simulink model "c_citation"  (R2020a)
settings: Solver=ode5  StartTime=0.0  StopTime=inf  FixedStep=0.01  RelTol=1e-3
InitFcn:
  | load('simulation_parameters');
values from neighbouring files (symbols this model uses):
  chord = 1.991    [citdata.mat]
  cv1 = 20000    [gear_params.m]
  cv2 = cv1    (= 20000)    [gear_params.m]
  cv3 = 4000    [gear_params.m]
  cv4 = 20000    [gear_params.m]
  deltagmax1 = 0.25    [gear_params.m]
  deltagmax2 = deltagmax1    (= 0.25)    [gear_params.m]
  deltagmax3 = 0.24    [gear_params.m]
  deltagmax4 = 0.02    [gear_params.m]
  ealphag = [0  0.2618  0.6981; 1  1.3  0.8]    [citdata.mat]
  ealphas = [0  0.2618  0.6981; 0.157  0.157  0.175]    [citdata.mat]
  g0 = 9.80665    [ac_genrl.mat]
  hDME = 0    [ac_genrl.mat]
  hGS = 0    [ac_genrl.mat]
  kt1 = 525020    [gear_params.m]
  kt2 = kt1    (= 525020)    [gear_params.m]
  kt3 = 457050    [gear_params.m]
  lh = 5.53    [citdata.mat]
  matbuaf = [0  -0.1745  0.4363; 0  -0.1  -0.1; 0.6981  -0.1  -0.1]    [citdata.mat]
  matdaf = [0 0 0.2618 0.6981 0.734842105263 0.771584210526 0.808326315789 0.845068421053 0.881810526316 0.918552631579 0.955294736842 0.992036842105 ... (529 elements, 23x23)]    [citdata.mat]
  matdam = [0 0.05 0.15 0.25 0.35 0.45 0.55 0.65 0.75 0.803571428571 0.857142857143 0.910714285714 ... (529 elements, 23x23)]    [citdata.mat]
  matdbbf = [0 0 0.6981 0.74464 0.79118 0.83772 0.88426 0.9308 0.97734 1.02388 1.07042 1.11696 ... (324 elements, 18x18)]    [citdata.mat]
  matdeaf = [0 0 0.2618 0.6981 0.734842105263 0.771584210526 0.808326315789 0.845068421053 0.881810526316 0.918552631579 0.955294736842 0.992036842105 ... (529 elements, 23x23)]    [citdata.mat]
  matdgaf = [0 0 0.2618 0.6981 -0.1745 -0.0175 -0.008 -0.009 0.4363 -0.0175 -0.008 -0.009 ... (16 elements, 4x4)]    [citdata.mat]
  matdqaf = [0 0 0.2618 0.6981 0.734842105263 0.771584210526 0.808326315789 0.845068421053 0.881810526316 0.918552631579 0.955294736842 0.992036842105 ... (529 elements, 23x23)]    [citdata.mat]
  matduaf = [0 0 0.2618 0.6981 0.734842105263 0.771584210526 0.808326315789 0.845068421053 0.881810526316 0.918552631579 0.955294736842 0.992036842105 ... (529 elements, 23x23)]    [citdata.mat]
  matdwaw = [0 0 0.1745 0.3491 0.5236 0.6458 1.2916 -0.1745 0 0.0018 0.0046 0.0088 ... (49 elements, 7x7)]    [citdata.mat]
  matedhr = [0 1 1 0.71 2 0.51 3 0.34 5 0.12 7.5 0.03 ... (20 elements, 2x10)]    [citdata.mat]
  mateif = [0  0.2618  0.6981; 0  -0.075  -0.075]    [citdata.mat]
  matelhr = [0 1 1 0.95 2 0.91 3 0.84 5 0.71 7.5 0.35 ... (20 elements, 2x10)]    [citdata.mat]
  matemhr = [0 1 1 0.9 2 0.8 3 0.7 5 0.5 7.5 0.25 ... (20 elements, 2x10)]    [citdata.mat]
  matemv1 = [0  90  100; 0  1  1]    [citdata.mat]
  matemv2 = [20  75  90; 0  1  1]    [citdata.mat]
  matemve = [0  90  100; 0  1  1]    [citdata.mat]
  matetam = [0  -0.1745  0.4363; 0  -0.04  -0.04; 1  -0.04  -0.04]    [citdata.mat]
  mateuaf = [0 0 0.6981 0.733005 0.76791 0.802815 0.83772 0.872625 0.90753 0.942435 0.97734 1.012245 ... (529 elements, 23x23)]    [citdata.mat]
  matfaaf = [0 0 0.2618 0.6981 0.734842105263 0.771584210526 0.808326315789 0.845068421053 0.881810526316 0.918552631579 0.955294736842 0.992036842105 ... (529 elements, 23x23)]    [citdata.mat]
  matfaxl = [0.15  0.35; 1  1]    [citdata.mat]
  matibaf = [0 0 0.2618 0.6981 -0.2 -0.119 -0.117 -0.108 0.3 -0.059 -0.052 -0.038 ... (16 elements, 4x4)]    [citdata.mat]
  matibb = [0 0 0.2618 1.571 3.142 -0.2 0 0 0.074 0.124 0 0 ... (50 elements, 5x10)]    [citdata.mat]
  matibmh = [0 0 15000 17142.8571429 19285.7142857 21428.5714286 23571.4285714 25714.2857143 27857.1428571 30000 0 0 ... (100 elements, 10x10)]    [citdata.mat]
  matipaf = [0  -0.1745  0.4363; 0  -0.44  -0.44; 0.6981  -0.44  -0.44]    [citdata.mat]
  matipmh = [0 0 15000 17142.8571429 19285.7142857 21428.5714286 23571.4285714 25714.2857143 27857.1428571 30000 0 0 ... (100 elements, 10x10)]    [citdata.mat]
  matiraf = [0 0 0.2618 0.6981 -0.2 0.05 -0.03 0.01 0.3 0.3 0.37 0.41 ... (16 elements, 4x4)]    [citdata.mat]
  matiuaf = [0  -0.2  0.3; 0  0.052  -0.003; 0.6981  0.052  -0.003]    [citdata.mat]
  matiwaf = [0  -0.1745  0.4363; 0  -0.185  -0.185; 0.6981  -0.185  -0.185]    [citdata.mat]
  matlaf = [0 0 0.2618 0.6981 0.734842105263 0.771584210526 0.808326315789 0.845068421053 0.881810526316 0.918552631579 0.955294736842 0.992036842105 ... (529 elements, 23x23)]    [citdata.mat]
  matlam = [0 0.05 0.15 0.25 0.35 0.45 0.55 0.65 0.75 0.803571428571 0.857142857143 0.910714285714 ... (529 elements, 23x23)]    [citdata.mat]
  matleaf = [0 0 0.2618 0.6981 0.734842105263 0.771584210526 0.808326315789 0.845068421053 0.881810526316 0.918552631579 0.955294736842 0.992036842105 ... (529 elements, 23x23)]    [citdata.mat]
  matleam = [0  -0.1745  0.4363; 0  0.58  0.58; 1  0.58  0.58]    [citdata.mat]
  matlgaf = [0 0 0.2618 0.6981 -0.1745 0.045 0.105 0.14 0.4363 0.045 0.105 0.14 ... (16 elements, 4x4)]    [citdata.mat]
  matlqaf = [0 0 0.2618 0.6981 0.734842105263 0.771584210526 0.808326315789 0.845068421053 0.881810526316 0.918552631579 0.955294736842 0.992036842105 ... (529 elements, 23x23)]    [citdata.mat]
  matluaf = [0 0 0.2618 0.6981 0.734842105263 0.771584210526 0.808326315789 0.845068421053 0.881810526316 0.918552631579 0.955294736842 0.992036842105 ... (529 elements, 23x23)]    [citdata.mat]
  matmaaf = [0 0 0.2618 0.6981 0.734842105263 0.771584210526 0.808326315789 0.845068421053 0.881810526316 0.918552631579 0.955294736842 0.992036842105 ... (484 elements, 22x22)]    [citdata.mat]
  matmaam = [0 0.05 0.15 0.25 0.35 0.45 0.55 0.65 0.75 0.803571428571 0.857142857143 0.910714285714 ... (484 elements, 22x22)]    [citdata.mat]
  matmaf = [0 0 0.2618 0.6981 0.734842105263 0.771584210526 0.808326315789 0.845068421053 0.881810526316 0.918552631579 0.955294736842 0.992036842105 ... (529 elements, 23x23)]    [citdata.mat]
  matmam = [0 0.05 0.15 0.25 0.35 0.45 0.55 0.65 0.75 0.803571428571 0.857142857143 0.910714285714 ... (529 elements, 23x23)]    [citdata.mat]
  matmbbf = [0 0 0.6981 0.74464 0.79118 0.83772 0.88426 0.9308 0.97734 1.02388 1.07042 1.11696 ... (324 elements, 18x18)]    [citdata.mat]
  matmeaf = [0 0 0.2618 0.6981 0.734842105263 0.771584210526 0.808326315789 0.845068421053 0.881810526316 0.918552631579 0.955294736842 0.992036842105 ... (529 elements, 23x23)]    [citdata.mat]
  matmeam = [0 0 1 1.05 1.1 1.15 1.2 1.25 1.3 1.35 1.4 1.45 ... (529 elements, 23x23)]    [citdata.mat]
  matmgaf = [0 0 0.2618 0.6981 -0.1745 -0.01 -0.024 -0.035 0.4363 -0.01 -0.024 -0.035 ... (16 elements, 4x4)]    [citdata.mat]
  matmqaf = [0 0 0.2618 0.6981 0.734842105263 0.771584210526 0.808326315789 0.845068421053 0.881810526316 0.918552631579 0.955294736842 0.992036842105 ... (529 elements, 23x23)]    [citdata.mat]
  matmrbr = [0  0  0.5236; 0  0  0; 0.384  0.001  0.001]    [citdata.mat]
  matnbab = [0 0 0.2618 1.571 3.142 -0.2 0 0 -0.0199 -0.1049 0 0 ... (25 elements, 5x5)]    [citdata.mat]
  matnbaf = [0  -0.2  0.3; 0  0.105  0.18; 0.6981  0.105  0.18]    [citdata.mat]
  matnbmh = [0 0 15000 17142.8571429 19285.7142857 21428.5714286 23571.4285714 25714.2857143 27857.1428571 30000 0 0 ... (100 elements, 10x10)]    [citdata.mat]
  matnpaf = [0 0 0.2618 0.6981 -0.2 0.03 0.03 0.05 0.3 -0.12 -0.12 -0.2 ... (16 elements, 4x4)]    [citdata.mat]
  matnpmh = [0 0 15000 17142.8571429 19285.7142857 21428.5714286 23571.4285714 25714.2857143 27857.1428571 30000 0 0 ... (100 elements, 10x10)]    [citdata.mat]
  matnraf = [0  -0.1745  0.4363; 0  -0.21  -0.21; 0.6981  -0.21  -0.21]    [citdata.mat]
  matnuaf = [0  -0.1745  0.4363; 0  -0.101  -0.101; 0.6981  -0.101  -0.101]    [citdata.mat]
  matnwaf = [0 0 0.2618 0.6981 -0.2 -0.02 -0.037 -0.049 0.3 0.03 0.043 0.036 ... (16 elements, 4x4)]    [citdata.mat]
  matnwmh = [0 0 15000 17142.8571429 19285.7142857 21428.5714286 23571.4285714 25714.2857143 27857.1428571 30000 0 0 ... (100 elements, 10x10)]    [citdata.mat]
  matqlaf = [0  -0.1745  0.4363; 0  -1  -1; 0.6981  -1  -1]    [citdata.mat]
  matquaf = [0 0 0.6981 0.733005 0.76791 0.802815 0.83772 0.872625 0.90753 0.942435 0.97734 1.012245 ... (529 elements, 23x23)]    [citdata.mat]
  matqxl = [0.15  0.35; 1  1]    [citdata.mat]
  matqxm = [0.15  0.35; 1  1]    [citdata.mat]
  matrtam = [0  -0.1745  0.4363; 0  0.011  0.011; 1  0.011  0.011]    [citdata.mat]
  matruaf = [0  -0.1745  0.4363; 0  0.2  0.2; 0.6981  0.2  0.2]    [citdata.mat]
  matrumh = [0 0 15000 17142.8571429 19285.7142857 21428.5714286 23571.4285714 25714.2857143 27857.1428571 30000 0 0 ... (100 elements, 10x10)]    [citdata.mat]
  matuut = [0  0.5  1; 0  1.35  1]    [citdata.mat]
  matwtam = [0  -0.1745  0.4363; 0  0.011  0.011; 1  0.011  0.011]    [citdata.mat]
  matybab = [0 0 0.2618 1.571 3.142 -0.2 0 0 0.34 0.75 0 0 ... (25 elements, 5x5)]    [citdata.mat]
  matybaf = [0  -0.1745  0.4363; 0  -0.75  -0.75; 0.6981  -0.75  -0.75]    [citdata.mat]
  matyraf = [0  -0.1745  0.4363; 0  0.85  0.85; 0.6981  0.85  0.85]    [citdata.mat]
  matyuaf = [0  -0.1745  0.4363; 0  0.23  0.23; 0.6981  0.23  0.23]    [citdata.mat]
  matywaf = [0  -0.1745  0.4363; 0  -0.04  -0.04; 0.6981  -0.04  -0.04]    [citdata.mat]
  murol = 0.03*10    (= 0.3)    [gear_params.m]
  P1 = 2000    [gear_params.m]
  P2 = P1    (= 2000)    [gear_params.m]
  P3 = 2550    [gear_params.m]
  P4 = 40000    [gear_params.m]
  psiLOC = 0    [ac_genrl.mat]
  pstat0 = 101325    [ac_genrl.mat]
  S = 24.99    [citdata.mat]
  span = 13.325    [citdata.mat]
  T0 = 288.15    [ac_genrl.mat]
  tilteng = [0 0]    [citdata.mat]
  toweng = [0 0]    [citdata.mat]
  vdommyr37 = [0  0.2618  0.6981; 0  0.025  0]    [citdata.mat]
  vdommyr38 = [0  0.2618  0.6981; -0.01  0  -0.01]    [citdata.mat]
  Vw915 = 0    [initcit.m]
  winddir = 45*(pi/180)    (= 0.785398163397)    [initcit.m]
  xcgref = 6.5    [citdata.mat]
  xDME = 0    [ac_genrl.mat]
  xeng = [8.407 8.407]    [citdata.mat]
  xGS = 0    [ac_genrl.mat]
  xiacc = 3.2    [ac_genrl.mat]
  xl1 = xcg-6.858    [gear_params.m]
  xl2 = xcg-6.858    [gear_params.m]
  xl3 = xcg-2.0752    [gear_params.m]
  xl4 = xcg-12.742    [gear_params.m]
  xLOC = 0    [ac_genrl.mat]
  ycgref = 0    [citdata.mat]
  yDME = 0    [ac_genrl.mat]
  yeng = [3 -3]    [citdata.mat]
  yGS = 0    [ac_genrl.mat]
  yiacc = 0    [ac_genrl.mat]
  yl1 = 1.918    [gear_params.m]
  yl2 = -1.918    [gear_params.m]
  yl3 = 0    [gear_params.m]
  ... (+9 more)
undefined symbols (not defined in the file or in its folder): Deng, massinit, matff, matn1d, matn2d, matthr, u0, ut0, x0, xt0
(part 1 of 5)
settings Model: ExtModeTrigMode=oneshot  ExtModeArmWhenConnect=off  Creator=laurensvaneykeren  LastModifiedBy=kdally
settings DataIOCC: SaveFormat=Array  SignalLoggingSaveFormat=ModelDataLogs  ReturnWorkspaceOutputs=off  SignalLoggingName=sigsOut
settings OptimizationCC: DefaultParameterBehavior=Inlined  UseDivisionForNetSlopeComputation=on  UseFloatMulNetSlope=on  InlineInvariantSignals=on  EnhancedBackFolding=on  PassReuseOutputArgsAs=Individual arguments  ExpressionDepthLimit=2147483647  ZeroExternalMemoryAtStartup=off  ZeroInternalMemoryAtStartup=off  NoFixptDivByZeroProtection=on  EfficientFloat2IntCast=on  OptimizeBlockOrder=speed  DifferentSizesBufferReuse=on  OptimizationCustomize=off  EfficientTunableParamExpr=on
settings DebuggingCC: ReadBeforeWriteMsg=EnableAllAsError  WriteAfterWriteMsg=EnableAllAsError  WriteAfterReadMsg=EnableAllAsError  SaveWithParameterizedLinksMsg=none  SignalResolutionControl=TryResolveAllWithWarning  MultiTaskRateTransMsg=warning  IntegerOverflowMsg=error  ParameterTunabilityLossMsg=error  FcnCallInpInsideContextMsg=warning  UniqueDataStoreMsg=error  StateNameClashWarn=warning  NonBusSignalsTreatedAsBus=error  SFInvalidInputDataAccessInChartInitDiag=error  SFTransitionOutsideNaturalParentDiag=error  SFUnreachableExecutionPathDiag=error  SFUndirectedBroadcastEventsDiag=error  SFExecutionAtInitializationDiag=none  IntegerSaturationMsg=error  ArithmeticOperatorsInVariantConditions=warning
settings HardwareCC: ProdBitPerLong=64  ProdHWDeviceType=Intel->x86-64 (Mac OS X)  TargetBitPerLong=64  TargetBitPerPointer=64  TargetBitPerSizeT=64  TargetBitPerPtrDiffT=64  TargetLongLongMode=on  TargetIntDivRoundTo=Zero  TargetEndianess=LittleEndian  TargetWordSize=64  TargetHWDeviceType=MATLAB Host  ProdEqTarget=off
settings SFSimCC: SimUseLocalCustomCode=off  MATLABDynamicMemAlloc=off  CustomCodeUndefinedFunction=UseInterfaceOnly
settings SFSimCC: SimCustomSourceCode=|
  | ac_axes.c
  | ac_atmos.c
settings RTWCC: SystemTargetFile=ert.tlc  GenCodeOnly=on  TemplateMakefile=ert_default_tmf  GenerateReport=on  RTWUseLocalCustomCode=off  BuildConfiguration=Faster Runs  IncludeHyperlinkInReport=on  LaunchReport=on  GenerateTraceInfo=on  GenerateTraceReport=on  GenerateTraceReportSl=on  GenerateTraceReportSf=on  GenerateTraceReportEml=on  GenerateCodeMetricsReport=on  CheckMdlBeforeBuild=Warning
settings CodeAppCC: ForceParamTrailComments=on  IgnoreCustomStorageClasses=off  OperatorAnnotations=on  SimulinkDataObjDesc=on  SFDataObjDesc=on  CustomSymbolStrGlobalVar=rt$N$M  CustomSymbolStrType=$N$M  CustomSymbolStrFcn=$N$M$F  CustomSymbolStrMacro=$N$M  InsertBlockDesc=on
settings ERTTargetCC: TargetLangStandard=C99 (ISO)  GenerateSampleERTMain=on  SupportAbsoluteTime=off  SupportComplex=off  SupportContinuousTime=on  SupportNonInlinedSFcns=on  InlinedParameterPlacement=NonHierarchical  ERTCustomFileTemplate=example_file_process.tlc
settings ConfigComp: CovMetricSettings=dw  CovHtmlReporting=on  CovSaveCumulativeToWorkspaceVar=on  CovSaveSingleToWorkspaceVar=on  CovExternalEMLEnable=off

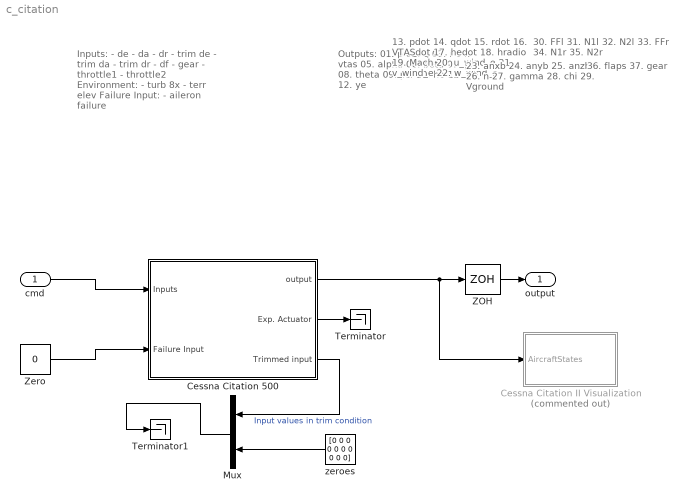
== system c_citation ==
  note: Inputs:
      |   - de
      |   - da
      |   - dr
      |   - trim de
      |   - trim da
      |   - trim dr
      |   - df
      |   - gear
      |   - throttle1
      |   - throttle2
      | Environment:
      |   - turb 8x
      |   - terr elev
      | Failure Input:
      |   - aileron failure
  note: Outputs:
      |   01. p
      |   02. q
      |   03. r
      |   04. vtas
      |   05. alpha
      |   06. beta
      |   07. phi
      |   08. theta
      |   09. psi
      |   10. he
      |   11. xe
      |   12. ye
  note: 13. pdot
      |   14. qdot
      |   15. rdot
      |   16. VTASdot
      |   17. hedot
      |   18. hradio
      |   19. Mach
      |   20. u_wind_e
      |   21. v_wind_e
      |   22. w_wind_e
  note: 23. anxb
      |   24. anyb
      |   25. anzb
      |   26. n
      |   27. gamma
      |   28. chi
      |   29. Vground
  note: 30. FFl
      |   31. N1l
      |   32. N2l
      |   33. FFr
      |   34. N1r
      |   35. N2r
  note: 36. flaps
      |   37. gear
  cmd : Inport  PortDimensions=10
  Cessna Citation 500 : Subsystem  mask(Citation Aircraft Model){trimdatafile=example.tri}
      mask prompts: trimdatafile "Trim Condition"
      mask init:
      | initcit;
      mask Display:
      | image(imread('Citation.jpg'))
      | port_label('input', 1, 'Inputs')
      | port_label('input', 2, 'Environment')
      | port_label('input', 3, 'Failure Input')
      | port_label('output', 1, 'Outputs')
      | port_label('output', 2, 'Exp. Actuator')
      | port_label('output', 3, 'Trim inputs')
  Cessna Citation II Visualization : Subsystem  Commented=on
  Mux : Mux  Inputs=2
  Terminator : Terminator
  Terminator1 : Terminator
  ZOH : ZeroOrderHold  SampleTime=-1
  Zero : Constant  Value=0  OutDataTypeStr=Inherit: Inherit via back propagation
  zeroes : Constant  Value=[0 0 0 0 0 0 0 0 0 0]  SampleTime=-1
  output : Outport  VectorParamsAs1DForOutWhenUnconnected=off
  wires:
  Cessna Citation 500/1(output) -> ZOH/1, Cessna Citation II Visualization/1(AircraftStates)
  Cessna Citation 500/3(Trimmed input) -> Mux/1  "Input values in trim condition"
  Cessna Citation 500/2(Exp. Actuator) -> Terminator/1
  cmd/1 -> Cessna Citation 500/1(Inputs)
  zeroes/1 -> Mux/2
  ZOH/1 -> output/1
  Zero/1 -> Cessna Citation 500/2(Failure Input)
  Mux/1 -> Terminator1/1

== system c_citation/Cessna Citation 500 ==
  note: p
      | q
      | r
      | vtas
      | alpha
      | beta
      | phi
      | theta
      | psi
      | he
      | xe
      | ye
  note: de
      | da
      | dr
      | dte
      | dta
      | dtr
      | df
      | gear
      | pla1
      | pla2
  note: pdot
      | qdot
      | rdot
      | VTASdot
      | hedot
  note: hradio
      | Mach
      | u_wind_e
      | v_wind_e
      | w_wind_e
  note: anxb
      | anyb
      | anzb
      | n
  note: gamma
      | chi
      | Vground
  note: turb 8x
      | terr_elev
  note: flaps
      | gear
  note: de
      | da
      | dr
      | dte
      | dta
      | dtr
      | df
      | gear
      | pla1
      | pla2
  note: FFl
      | N1l
      | N2l
      | FFr
      | N1r
      | N2r
  Inputs : Inport
  Failure Input : Inport  Port=2
  Actuators : Subsystem
  Citation model DASMAT : Subsystem
  Controllers : Subsystem
  Demux4 : Demux  Outputs=[8 2]
      settings: DisplayOption=none
  Mux1 : Mux  Inputs=7
  Mux2 : Mux  Inputs=2
  Terminator : Terminator
  Vector Concatenate : Concatenate  NumInputs=9
  Zero1 : Constant  Value=0  OutDataTypeStr=Inherit: Inherit via back propagation
  trim conditions : Subsystem
  ua sel : Selector  IndexOptions=Index vector (dialog)  Indices=[5 6]  OutputSizes=1
  xdot sel : Selector  IndexOptions=Index vector (dialog)  Indices=[1 2 3 4 10]  OutputSizes=1
  yacc sel : Selector  IndexOptions=Index vector (dialog)  Indices=[4 5 6 15]  OutputSizes=1
  yair sel : Selector  IndexOptions=Index vector (dialog)  Indices=[6 9 22 23 24]  OutputSizes=1
  yfp sel : Selector  IndexOptions=Index vector (dialog)  Indices=[1 2 15]  OutputSizes=1
  ypp sel : Selector  IndexOptions=Index vector (dialog)  Indices=[2 3 4 13 14 15]  OutputSizes=1
  output : Outport  PortDimensions=12  VectorParamsAs1DForOutWhenUnconnected=off
  Exp. Actuator : Outport  Port=2  VectorParamsAs1DForOutWhenUnconnected=off
  Trimmed input : Outport  Port=3  VectorParamsAs1DForOutWhenUnconnected=off
  wires:
  Inputs/1 -> Controllers/2(inputs)
  Demux4/1 -> Citation model DASMAT/1(ua), ua sel/1
  Demux4/2 -> Citation model DASMAT/2(ut)
  Citation model DASMAT/3(yair) -> yair sel/1
  yair sel/1 -> Mux1/3
  Citation model DASMAT/2(xdot) -> xdot sel/1
  xdot sel/1 -> Mux1/2
  yacc sel/1 -> Mux1/4
  Citation model DASMAT/4(yacc) -> yacc sel/1
  yfp sel/1 -> Mux1/5
  Citation model DASMAT/5(yfp) -> yfp sel/1
  Actuators/1(Out) -> Demux4/1
  trim conditions/1(ua) -> Mux2/1
  trim conditions/2(ut) -> Mux2/2
  Mux2/1 -> Trimmed input/1
  Controllers/1(control inputs) -> Actuators/1(In)
  ua sel/1 -> Mux1/7
  Citation model DASMAT/6(ypp) -> ypp sel/1
  ypp sel/1 -> Mux1/6
  Failure Input/1 -> Actuators/2(failure)
  Actuators/2(Expected) -> Exp. Actuator/1
  Citation model DASMAT/1(x) -> output/1, Mux1/1, Controllers/1(state)
  Mux1/1 -> Terminator/1
  Zero1/1 -> Vector Concatenate/2, Vector Concatenate/1, Vector Concatenate/4, Vector Concatenate/6, Vector Concatenate/5, Vector Concatenate/3, Vector Concatenate/9, Vector Concatenate/8, Vector Concatenate/7
  Vector Concatenate/1 -> Citation model DASMAT/3(Environment)

== system c_citation/Cessna Citation II Visualization ==
  AircraftStates : Inport
  1 : Terminator
  2 : Terminator
  3D Display : Subsystem
  Alt < 10 m => Stop : Fcn  Expr=u<10
  Demux1 : Demux  Outputs=[6 1 1 1 1 27]
      settings: DisplayOption=none
  Stop Simulation : Stop
  wires:
  AircraftStates/1 -> Demux1/1
  Demux1/1 -> 1/1
  Demux1/5 -> Alt < 10 m => Stop/1
  Demux1/2 -> 3D Display/1(roll)
  Demux1/3 -> 3D Display/2(pitch)
  Demux1/4 -> 3D Display/3(yaw)
  Demux1/6 -> 2/1
  Alt < 10 m => Stop/1 -> Stop Simulation/1

== system c_citation/Cessna Citation 500/Actuators ==
  note: Expected control deflections
  note: Add failure to aileron channel
  note: de
      | da
      | dr
      | dte
      | dta
      | dtr
      | df
      | gear
      | pla1
      | pla2
  note: de
      | da
      | dr
      | dte
      | dta
      | dtr
      | df
      | gear
      | pla1
      | pla2
  In : Inport
  failure : Inport  Port=2
  Demux : Demux  Outputs=10
      settings: DisplayOption=none
  Demux1 : Demux  Outputs=[1 1 8]
  Gain : Gain  Gain=0.5
  Mux : Mux  Inputs=10
  Mux1 : Mux  Inputs=3
  Product : Product
  Sum : Sum  Inputs=+-|
  Sum1 : Sum  Inputs=++|
  da : Subsystem  Commented=through
  da limits : Saturate  UpperLimit=0.65  LowerLimit=-0.65
  de : Subsystem  Commented=through
  de limits : Saturate  UpperLimit=0.26  LowerLimit=-0.35
  dr : Subsystem  Commented=through
  dr limits : Saturate  UpperLimit=0.38  LowerLimit=-0.38
  failure angle left aileron : Constant  Value=0.28
  flaps : Subsystem  Commented=through
  gear : Subsystem  Commented=through
  Out : Outport  VectorParamsAs1DForOutWhenUnconnected=off
  Expected : Outport  Port=2  VectorParamsAs1DForOutWhenUnconnected=off
  wires:
  In/1 -> Demux/1
  Demux/1 -> de/1(In)
  Demux/2 -> da/1(In)
  Demux/3 -> dr/1(In)
  de/1(Out) -> de limits/1
  da/1(Out) -> da limits/1
  da limits/1 -> Mux/2, Gain/1
  dr/1(Out) -> dr limits/1
  dr limits/1 -> Mux/3
  de limits/1 -> Mux/1
  Demux/8 -> gear/1(In)
  Demux/7 -> flaps/1(In)
  Demux/9 -> Mux/9
  Demux/10 -> Mux/10
  flaps/1(Out) -> Mux/7
  gear/1(Out) -> Mux/8
  Demux/4 -> Mux/4
  Demux/5 -> Mux/5
  Demux/6 -> Mux/6
  failure angle left aileron/1 -> Sum/1
  Gain/1 -> Sum/2
  Sum/1 -> Product/2
  failure/1 -> Product/1
  Mux/1 -> Expected/1, Demux1/1
  Mux1/1 -> Out/1
  Demux1/1 -> Mux1/1
  Demux1/3 -> Mux1/3
  Demux1/2 -> Sum1/2
  Sum1/1 -> Mux1/2
  Product/1 -> Sum1/1

== system c_citation/Cessna Citation 500/Citation model DASMAT ==
  ua : Inport
  ut : Inport  Port=2
  Environment : Inport  Port=3
  AIRCRAFT MODEL : Subsystem
  Mux1 : Mux  Inputs=[8 2 8 12 8]
  Terminator_{16..19} (4 alike) : Terminator
  massinit : Constant  Value=massinit
  x : Outport  VectorParamsAs1DForOutWhenUnconnected=off
  xdot : Outport  Port=2  VectorParamsAs1DForOutWhenUnconnected=off
  yair : Outport  Port=3  VectorParamsAs1DForOutWhenUnconnected=off
  yacc : Outport  Port=4  VectorParamsAs1DForOutWhenUnconnected=off
  yfp : Outport  Port=5  VectorParamsAs1DForOutWhenUnconnected=off
  ypp : Outport  Port=6  VectorParamsAs1DForOutWhenUnconnected=off
  wires:
  AIRCRAFT MODEL/13(FMt) -> Terminator_19/1
  Mux1/1 -> yair/1
  AIRCRAFT MODEL/12(FMag) -> Terminator_17/1
  AIRCRAFT MODEL/11(FMa) -> Terminator_18/1
  AIRCRAFT MODEL/7(gust) -> Mux1/5
  AIRCRAFT MODEL/6(wind) -> Mux1/4
  AIRCRAFT MODEL/5(yad2) -> Mux1/3
  AIRCRAFT MODEL/4(yad1) -> Mux1/2
  AIRCRAFT MODEL/3(yatm) -> Mux1/1
  AIRCRAFT MODEL/2(xdot) -> xdot/1
  AIRCRAFT MODEL/1(x) -> x/1
  AIRCRAFT MODEL/10(ys) -> Terminator_16/1
  AIRCRAFT MODEL/9(yfp) -> yfp/1
  AIRCRAFT MODEL/8(yacc) -> yacc/1
  massinit/1 -> AIRCRAFT MODEL/3(massinit)
  ut/1 -> AIRCRAFT MODEL/2(ut)
  ua/1 -> AIRCRAFT MODEL/1(ua)
  Environment/1 -> AIRCRAFT MODEL/4(Environment)
  AIRCRAFT MODEL/14(ypp) -> ypp/1

== system c_citation/Cessna Citation 500/Controllers ==
  state : Inport
  inputs : Inport  Port=2
  A/T enabled : Gain  SaturateOnIntegerOverflow=on  OutDataTypeStr=Inherit: Same as input  ParamDataTypeStr=Inherit: Same as input
  Yaw damper : Subsystem
  add controller outputs to pilot inputs : Sum  Inputs=|+|+|+|  SaturateOnIntegerOverflow=on
  auto throttle : Subsystem
  control inputs : Outport  VectorParamsAs1DForOutWhenUnconnected=off
  wires:
  state/1 -> Yaw damper/1(state), auto throttle/1(state)
  inputs/1 -> Yaw damper/2(inputs), add controller outputs to pilot inputs/3, auto throttle/2(inputs)
  add controller outputs to pilot inputs/1 -> control inputs/1
  Yaw damper/1(controller output) -> add controller outputs to pilot inputs/1
  auto throttle/1(controller output) -> A/T enabled/1
  A/T enabled/1 -> add controller outputs to pilot inputs/2

== system c_citation/Cessna Citation 500/trim conditions ==
  PLA1/Tx1 : Constant  Value=ut0(1)
  PLA2/Tx2 : Constant  Value=ut0(2)
  control inputs : Mux  Inputs=8
      settings: DisplayOption=signals
  deltaa : Constant  Value=u0(2)
  deltae : Constant  Value=u0(1)
  deltaf : Constant  Value=u0(7)
  deltar : Constant  Value=u0(3)
  deltata : Constant  Value=u0(5)
  deltate : Constant  Value=u0(4)
  deltatr : Constant  Value=u0(6)
  engine inputs : Mux  Inputs=2
      settings: DisplayOption=signals
  lgsw : Constant  Value=u0(8)
  ua : Outport  VectorParamsAs1DForOutWhenUnconnected=off
  ut : Outport  Port=2  VectorParamsAs1DForOutWhenUnconnected=off
  wires:
  deltaf/1 -> control inputs/7  "df"
  engine inputs/1 -> ut/1
  deltatr/1 -> control inputs/6  "dtr"
  deltata/1 -> control inputs/5  "dta"
  control inputs/1 -> ua/1
  PLA1/Tx1/1 -> engine inputs/1  "pla1"
  PLA2/Tx2/1 -> engine inputs/2  "pla2"
  deltae/1 -> control inputs/1  "de"
  deltaa/1 -> control inputs/2  "da"
  deltar/1 -> control inputs/3  "dr"
  deltate/1 -> control inputs/4  "dte"
  lgsw/1 -> control inputs/8  "lg"

== system c_citation/Cessna Citation II Visualization/3D Display ==
  roll : Inport
  pitch : Inport  Port=2
  yaw : Inport  Port=3
  Mux1 : Mux
  Position : Subsystem
  S-Function : S-Function  FunctionName=cessnac550_3d_sfnc  SFunctionDeploymentMode=off  EnableBusSupport=off
  Stop Simulation : Stop
  wires:
  roll/1 -> Mux1/1
  Position/1(Out1) -> Mux1/4
  pitch/1 -> Mux1/2
  yaw/1 -> Mux1/3
  Mux1/1 -> S-Function/1
  S-Function/1 -> Stop Simulation/1

== system c_citation/Cessna Citation 500/Actuators/da ==
  In : Inport
  Gain : Gain  Gain=13  SaturateOnIntegerOverflow=on  OutDataTypeStr=Inherit: Same as input  ParamDataTypeStr=Inherit: Same as input
  Integrator : Integrator  InitialCondition=u0(2)
  Sum : Sum  Inputs=|+-  SaturateOnIntegerOverflow=on
  Out : Outport  VectorParamsAs1DForOutWhenUnconnected=off
  wires:
  Integrator/1 -> Out/1, Sum/2
  In/1 -> Sum/1
  Sum/1 -> Gain/1
  Gain/1 -> Integrator/1

== system c_citation/Cessna Citation 500/Actuators/de ==
  In : Inport
  Gain : Gain  Gain=13  SaturateOnIntegerOverflow=on  OutDataTypeStr=Inherit: Same as input  ParamDataTypeStr=Inherit: Same as input
  Integrator : Integrator  InitialCondition=u0(1)
  Sum : Sum  Inputs=|+-  SaturateOnIntegerOverflow=on
  Out : Outport  VectorParamsAs1DForOutWhenUnconnected=off
  wires:
  Integrator/1 -> Out/1, Sum/2
  In/1 -> Sum/1
  Sum/1 -> Gain/1
  Gain/1 -> Integrator/1

== system c_citation/Cessna Citation 500/Actuators/dr ==
  In : Inport
  Gain : Gain  Gain=13  SaturateOnIntegerOverflow=on  OutDataTypeStr=Inherit: Same as input  ParamDataTypeStr=Inherit: Same as input
  Integrator : Integrator  InitialCondition=u0(3)
  Sum : Sum  Inputs=|+-  SaturateOnIntegerOverflow=on
  Out : Outport  VectorParamsAs1DForOutWhenUnconnected=off
  wires:
  Integrator/1 -> Out/1, Sum/2
  In/1 -> Sum/1
  Sum/1 -> Gain/1
  Gain/1 -> Integrator/1

== system c_citation/Cessna Citation 500/Actuators/flaps ==
  In : Inport
  Gain : Gain  Gain=0.9  SaturateOnIntegerOverflow=on  OutDataTypeStr=Inherit: Same as input  ParamDataTypeStr=Inherit: Same as input
  Integrator : Integrator  InitialCondition=u0(7)
  Sum : Sum  Inputs=|+-  SaturateOnIntegerOverflow=on
  Out : Outport  VectorParamsAs1DForOutWhenUnconnected=off
  wires:
  Integrator/1 -> Out/1, Sum/2
  In/1 -> Sum/1
  Sum/1 -> Gain/1
  Gain/1 -> Integrator/1

== system c_citation/Cessna Citation 500/Actuators/gear ==
  In : Inport
  Gain : Gain  Gain=0.6  SaturateOnIntegerOverflow=on  OutDataTypeStr=Inherit: Same as input  ParamDataTypeStr=Inherit: Same as input
  Integrator : Integrator  InitialCondition=u0(8)
  Sum : Sum  Inputs=|+-  SaturateOnIntegerOverflow=on
  Out : Outport  VectorParamsAs1DForOutWhenUnconnected=off
  wires:
  Integrator/1 -> Out/1, Sum/2
  In/1 -> Sum/1
  Sum/1 -> Gain/1
  Gain/1 -> Integrator/1

== system c_citation/Cessna Citation 500/Citation model DASMAT/AIRCRAFT MODEL ==
  ua : Inport
  ut : Inport  Port=2
  massinit : Inport  Port=3
  Environment : Inport  Port=4
  AFM : Subsystem
  AIRDATA : Subsystem
  Demux : Demux  Outputs=[8 1]
      settings: DisplayOption=none
  EFM : Subsystem
  EQM : Subsystem
  FM SORT : Subsystem
  GRAVITY : Subsystem
  LANDING GEAR : Subsystem
  OBSERVATIONS : Subsystem
  WIND/TURBULENCE : Subsystem
  x : Outport  VectorParamsAs1DForOutWhenUnconnected=off
  xdot : Outport  Port=2  VectorParamsAs1DForOutWhenUnconnected=off
  yatm : Outport  Port=3  VectorParamsAs1DForOutWhenUnconnected=off
  yad1 : Outport  Port=4  VectorParamsAs1DForOutWhenUnconnected=off
  yad2 : Outport  Port=5  VectorParamsAs1DForOutWhenUnconnected=off
  wind : Outport  Port=6  VectorParamsAs1DForOutWhenUnconnected=off
  gust : Outport  Port=7  VectorParamsAs1DForOutWhenUnconnected=off
  yacc : Outport  Port=8  VectorParamsAs1DForOutWhenUnconnected=off
  yfp : Outport  Port=9  VectorParamsAs1DForOutWhenUnconnected=off
  ys : Outport  Port=10  VectorParamsAs1DForOutWhenUnconnected=off
  FMa : Outport  Port=11  VectorParamsAs1DForOutWhenUnconnected=off
  FMag : Outport  Port=12  VectorParamsAs1DForOutWhenUnconnected=off
  FMt : Outport  Port=13  VectorParamsAs1DForOutWhenUnconnected=off
  ypp : Outport  Port=14  VectorParamsAs1DForOutWhenUnconnected=off
  wires:
  AFM/1(FMa) -> FM SORT/1(FMa), EQM/2(FMa)
  OBSERVATIONS/3(ys) -> ys/1
  OBSERVATIONS/2(yfp) -> yfp/1
  EQM/4(FMtot corrected) -> OBSERVATIONS/4(FMtot)
  EQM/3(yuvw) -> OBSERVATIONS/3(yuvw)
  EFM/1(FMt) -> FM SORT/3(FMt), FMt/1
  AFM/4(FMag) -> FM SORT/2(FMag), FMag/1
  ua/1 -> AFM/2(ua), LANDING GEAR/4(ua)
  ut/1 -> EFM/2(ut)
  OBSERVATIONS/1(yacc) -> yacc/1
  FM SORT/1(FMtot) -> EQM/1("FMtot ")
  EQM/5(FMa corrected) -> OBSERVATIONS/5(FMa), FMa/1
  AFM/2(FMadot) -> EQM/3(FMadot)
  AFM/3(FMbdot) -> EQM/4(FMbdot)
  GRAVITY/1(Fgr) -> FM SORT/4("Fgr "), OBSERVATIONS/6(Fgr)
  massinit/1 -> EFM/3(massinit), AFM/3(massinit), GRAVITY/2(massinit), EQM/5(massinit), OBSERVATIONS/7(massinit), LANDING GEAR/3(massinit)
  AIRDATA/3(yad2) -> EFM/6(yad2), AFM/5(yad2), yad2/1
  AIRDATA/2(yad1) -> AFM/4(yad1), EFM/5(yad1), yad1/1
  AIRDATA/1(yatm) -> yatm/1, GRAVITY/3(yatm), OBSERVATIONS/8(yatm), EFM/4(yatm), AFM/7(yatm)
  EQM/1(x) -> GRAVITY/1("x "), LANDING GEAR/1(x), EFM/1(x), AFM/1(x), WIND/TURBULENCE/1("x "), AIRDATA/1(x), x/1, OBSERVATIONS/1(x)
  WIND/TURBULENCE/1(wind) -> EQM/6(wind), wind/1
  EQM/2(xdot) -> xdot/1, OBSERVATIONS/2(xdot), LANDING GEAR/2(xdot)
  Environment/1 -> Demux/1
  Demux/1 -> gust/1, AFM/6(gust)
  Demux/2 -> AIRDATA/2(terrain elevation), LANDING GEAR/5(terr elev)  "terrain elevation"
  LANDING GEAR/1(Fmt) -> FM SORT/5(Fgear)
  EFM/2(ypp) -> ypp/1

== system c_citation/Cessna Citation 500/Controllers/Yaw damper ==
  state : Inport
  inputs : Inport  Port=2
  Gain : Gain  SaturateOnIntegerOverflow=on  OutDataTypeStr=Inherit: Same as input  ParamDataTypeStr=Inherit: Same as input
  Washout : TransferFcn  Numerator=[1 0]  Denominator=[1 1/4]
  dr : Gain  Gain=[0 0 1 0 0 0 0 0 0 0]  SaturateOnIntegerOverflow=on  OutDataTypeStr=Inherit: Same as input  ParamDataTypeStr=Inherit: Same as input
  not used : Terminator
  r  sel : Selector  IndexOptions=Index vector (dialog)  Indices=[3]  OutputSizes=1
  controller output : Outport  VectorParamsAs1DForOutWhenUnconnected=off
  wires:
  Washout/1 -> Gain/1
  dr/1 -> controller output/1
  state/1 -> r  sel/1
  r  sel/1 -> Washout/1  "r"
  inputs/1 -> not used/1
  Gain/1 -> dr/1

== system c_citation/Cessna Citation 500/Controllers/auto throttle ==
  state : Inport
  inputs : Inport  Port=2
  Gain : Gain  Gain=0.5  SaturateOnIntegerOverflow=on  OutDataTypeStr=Inherit: Same as input  ParamDataTypeStr=Inherit: Same as input
  Saturation : Saturate  UpperLimit=1.0  LowerLimit=0.0
  Sum : Sum  Inputs=+-|  SaturateOnIntegerOverflow=on
  VTAS ref (trim value) : Constant  Value=x0(4)
  VTAS sel : Selector  IndexOptions=Index vector (dialog)  Indices=[4]  OutputSizes=1
  controller output is later added to pilot input! : Sum  Inputs=|+-  SaturateOnIntegerOverflow=on
  pla1&2 : Gain  Gain=[0 0 0 0 0 0 0 0 1 1]  SaturateOnIntegerOverflow=on  OutDataTypeStr=Inherit: Same as input  ParamDataTypeStr=Inherit: Same as input
  pla1&2 as well : Gain  Gain=[0 0 0 0 0 0 0 0 1 1]  SaturateOnIntegerOverflow=on  OutDataTypeStr=Inherit: Same as input  ParamDataTypeStr=Inherit: Same as input
  controller output : Outport  VectorParamsAs1DForOutWhenUnconnected=off
  wires:
  inputs/1 -> pla1&2 as well/1
  state/1 -> VTAS sel/1
  VTAS sel/1 -> Sum/2  "VTAS"
  VTAS ref (trim value)/1 -> Sum/1
  Sum/1 -> Gain/1
  pla1&2/1 -> controller output is later added to pilot input!/1
  Gain/1 -> Saturation/1
  controller output is later added to pilot input!/1 -> controller output/1
  Saturation/1 -> pla1&2/1
  pla1&2 as well/1 -> controller output is later added to pilot input!/2

== system c_citation/Cessna Citation II Visualization/3D Display/Position ==
  Mux2 : Mux  Inputs=3
  x : Constant  Value=0
  y : Constant  Value=0
  z : Constant  Value=0
  Out1 : Outport  VectorParamsAs1DForOutWhenUnconnected=off
  wires:
  y/1 -> Mux2/2
  z/1 -> Mux2/3
  x/1 -> Mux2/1
  Mux2/1 -> Out1/1

== system c_citation/Cessna Citation 500/Citation model DASMAT/AIRCRAFT MODEL/AFM ==
  x : Inport
  ua : Inport  Port=2
  massinit : Inport  Port=3
  yad1 : Inport  Port=4
  yad2 : Inport  Port=5
  gust : Inport  Port=6
  yatm : Inport  Port=7
  Aero axes-cg transformation : Subsystem
  Aeromod : Subsystem
  FMaerodims : Subsystem
  FMgustdims : Subsystem
  Gust axes-cg transformation : Subsystem
  FMa : Outport  VectorParamsAs1DForOutWhenUnconnected=off
  FMadot : Outport  Port=2  VectorParamsAs1DForOutWhenUnconnected=off
  FMbdot : Outport  Port=3  VectorParamsAs1DForOutWhenUnconnected=off
  FMag : Outport  Port=4  VectorParamsAs1DForOutWhenUnconnected=off
  wires:
  FMaerodims/3(FMbdot) -> FMbdot/1
  FMgustdims/1(FMag) -> FMag/1
  FMaerodims/2(FMadot) -> FMadot/1
  FMaerodims/1(FMa) -> FMa/1
  ua/1 -> Aeromod/2(ua)
  yad2/1 -> Aeromod/5(yad2)
  gust/1 -> Aeromod/6(gust)
  Aero axes-cg transformation/1(Ca) -> FMaerodims/1(Ca)
  Aero axes-cg transformation/2(Cadot) -> FMaerodims/2(Cadot)
  Aero axes-cg transformation/3(Cbdot) -> FMaerodims/3(Cbdot)
  Gust axes-cg transformation/1(Cag) -> FMgustdims/1(Cag)
  yad1/1 -> FMaerodims/5(yad1), FMgustdims/2(yad1), Aeromod/4(yad1)
  massinit/1 -> Aero axes-cg transformation/5(massinit), Gust axes-cg transformation/3(massinit), Aeromod/3(massinit)
  Aeromod/1(Ca) -> Aero axes-cg transformation/1(Ca model)
  Aeromod/2(Cadot) -> Aero axes-cg transformation/2(Cadot model)
  Aeromod/3(Cbdot) -> Aero axes-cg transformation/3(Cbdot model)
  Aeromod/4(Cag) -> Gust axes-cg transformation/1(Cag model)
  x/1 -> Aero axes-cg transformation/4("x "), Gust axes-cg transformation/2("x "), FMaerodims/4(x), Aeromod/1(x)
  yatm/1 -> Aeromod/7(yatm)

== system c_citation/Cessna Citation 500/Citation model DASMAT/AIRCRAFT MODEL/AIRDATA ==
  x : Inport
  terrain elevation : Inport  Port=2
  Demux : Demux  Outputs=[8 2 8]
      settings: DisplayOption=none
  Demux1 : Demux  Outputs=[5 1 2]
      settings: DisplayOption=none
  Mux : Mux  Inputs=[5 1 2]
  Sum : Sum  Inputs=-+|  SaturateOnIntegerOverflow=on
  airdata : S-Function  FunctionName=ac_atmos  SFunctionDeploymentMode=off  EnableBusSupport=off
  yatm : Outport  VectorParamsAs1DForOutWhenUnconnected=off
  yad1 : Outport  Port=2  VectorParamsAs1DForOutWhenUnconnected=off
  yad2 : Outport  Port=3  VectorParamsAs1DForOutWhenUnconnected=off
  wires:
  x/1 -> airdata/1
  airdata/1 -> Demux/1
  Demux/2 -> yad1/1
  Demux/3 -> yad2/1
  Demux/1 -> Demux1/1
  Mux/1 -> yatm/1
  Demux1/1 -> Mux/1
  Demux1/3 -> Mux/3
  Demux1/2 -> Sum/2
  Sum/1 -> Mux/2
  terrain elevation/1 -> Sum/1

== system c_citation/Cessna Citation 500/Citation model DASMAT/AIRCRAFT MODEL/EFM ==
  x : Inport
  ut : Inport  Port=2
  massinit : Inport  Port=3
  yatm : Inport  Port=4
  yad1 : Inport  Port=5
  yad2 : Inport  Port=6
  Engine axes-cg transformation : Subsystem
  Engmod : Subsystem
  FMt : Outport  VectorParamsAs1DForOutWhenUnconnected=off
  ypp : Outport  Port=2  VectorParamsAs1DForOutWhenUnconnected=off
  wires:
  massinit/1 -> Engine axes-cg transformation/3(massinit)
  Engine axes-cg transformation/1(FMt) -> FMt/1
  ut/1 -> Engmod/2(ut)
  yatm/1 -> Engmod/3(yatm)
  yad2/1 -> Engmod/5(yad2)
  x/1 -> Engine axes-cg transformation/2("x "), Engmod/1(x)
  yad1/1 -> Engmod/4(yad1)
  Engmod/1(FMt) -> Engine axes-cg transformation/1(FMt model)
  Engmod/2(ypp) -> ypp/1

== system c_citation/Cessna Citation 500/Citation model DASMAT/AIRCRAFT MODEL/EQM ==
  "FMtot " : Inport
  FMa : Inport  Port=2
  FMadot : Inport  Port=3
  FMbdot : Inport  Port=4
  massinit : Inport  Port=5
  wind : Inport  Port=6
  CFMa correction : Subsystem
  Integrator : Integrator  InitialCondition=x0
  State Derivatives : Subsystem
  x : Outport  VectorParamsAs1DForOutWhenUnconnected=off
  xdot : Outport  Port=2  VectorParamsAs1DForOutWhenUnconnected=off
  yuvw : Outport  Port=3  VectorParamsAs1DForOutWhenUnconnected=off
  FMtot corrected : Outport  Port=4  VectorParamsAs1DForOutWhenUnconnected=off
  FMa corrected : Outport  Port=5  VectorParamsAs1DForOutWhenUnconnected=off
  wires:
  State Derivatives/2(yuvw) -> yuvw/1
  State Derivatives/3(FMtot corrected) -> FMtot corrected/1
  FMa/1 -> CFMa correction/2(FMa)
  State Derivatives/1(xdot) -> xdot/1, CFMa correction/1(xdot), Integrator/1
  CFMa correction/1(FMa corrected) -> FMa corrected/1
  massinit/1 -> State Derivatives/5(massinit)
  "FMtot "/1 -> State Derivatives/2(FMtot)
  FMadot/1 -> CFMa correction/3(FMadot), State Derivatives/3(FMadot)
  FMbdot/1 -> CFMa correction/4(FMbdot), State Derivatives/4(FMbdot)
  Integrator/1 -> State Derivatives/1(x), x/1
  wind/1 -> State Derivatives/6(wind)

== system c_citation/Cessna Citation 500/Citation model DASMAT/AIRCRAFT MODEL/FM SORT ==
  FMa : Inport
  FMag : Inport  Port=2
  FMt : Inport  Port=3
  "Fgr " : Inport  Port=4
  Fgear : Inport  Port=5
  Mux : Mux  Inputs=[12 12]
  Sum : Sum  Inputs=+++++  InputSameDT=on  SaturateOnIntegerOverflow=on  OutDataTypeStr=Inherit: Same as first input
  Sum1 : Sum  Inputs=++++  InputSameDT=on  SaturateOnIntegerOverflow=on  OutDataTypeStr=Inherit: Same as first input
  aero : Demux  Outputs=[12 12]
      settings: DisplayOption=none
  engine : Demux  Outputs=[12 12]
      settings: DisplayOption=none
  gear : Demux  Outputs=[12 12]
      settings: DisplayOption=none
  gust : Demux  Outputs=[12 12]
      settings: DisplayOption=none
  FMtot : Outport  VectorParamsAs1DForOutWhenUnconnected=off
  wires:
  FMt/1 -> engine/1
  FMa/1 -> aero/1
  FMag/1 -> gust/1
  gust/2 -> Sum1/2
  Sum1/1 -> Mux/2
  engine/2 -> Sum1/3
  aero/2 -> Sum1/1
  gust/1 -> Sum/2
  engine/1 -> Sum/3
  Sum/1 -> Mux/1
  "Fgr "/1 -> Sum/4
  aero/1 -> Sum/1
  Mux/1 -> FMtot/1
  Fgear/1 -> gear/1
  gear/1 -> Sum/5
  gear/2 -> Sum1/4

== system c_citation/Cessna Citation 500/Citation model DASMAT/AIRCRAFT MODEL/GRAVITY ==
  "x " : Inport
  massinit : Inport  Port=2
  yatm : Inport  Port=3
  Fgr transformation : S-Function  FunctionName=ac_axes  Parameters=3  SFunctionDeploymentMode=off  EnableBusSupport=off
  Mux : Mux  Inputs=[12 3]
  Mux1 : Mux  Inputs=3
  Terminator_{1..9} (9 alike) : Terminator
  W : Product  InputSameDT=on  SaturateOnIntegerOverflow=on  OutDataTypeStr=Inherit: Same as first input
  atmosphere : Demux  Outputs=8
      settings: DisplayOption=none
  mass cg inertia : Demux  Outputs=[1 3 4]
      settings: DisplayOption=none
  zero : Constant  Value=0
  Fgr : Outport  VectorParamsAs1DForOutWhenUnconnected=off
  wires:
  mass cg inertia/3 -> Terminator_9/1
  mass cg inertia/2 -> Terminator_8/1
  atmosphere/8 -> Terminator_7/1
  atmosphere/7 -> Terminator_6/1
  atmosphere/6 -> Terminator_5/1
  atmosphere/5 -> Terminator_4/1
  atmosphere/3 -> Terminator_3/1
  atmosphere/2 -> Terminator_2/1
  atmosphere/1 -> Terminator_1/1
  Mux/1 -> Fgr transformation/1
  "x "/1 -> Mux/1
  Fgr transformation/1 -> Fgr/1
  mass cg inertia/1 -> W/1
  massinit/1 -> mass cg inertia/1
  yatm/1 -> atmosphere/1
  W/1 -> Mux1/3
  Mux1/1 -> Mux/2
  zero/1 -> Mux1/1, Mux1/2
  atmosphere/4 -> W/2

== system c_citation/Cessna Citation 500/Citation model DASMAT/AIRCRAFT MODEL/LANDING GEAR ==
  note: Landing Gear Model
      | Cessna Citation 500
      | Version 0.04NLR
      | (c) A.R. Veldhuijzen September 2001
  x : Inport
  xdot : Inport  Port=2
  massinit : Inport  Port=3
  ua : Inport  Port=4
  terr elev : Inport  Port=5
  Gear axes-cg transformation : Subsystem
  Landing Gear model : Subsystem
  Switch : Switch  Threshold=0.95  SaturateOnIntegerOverflow=on
  gear position : Selector  IndexOptions=Index vector (dialog)  Indices=[8]  OutputSizes=1
  zero : Constant  Value=[0 0 0 0 0 0]
  Fmt : Outport  VectorParamsAs1DForOutWhenUnconnected=off
  wires:
  xdot/1 -> Landing Gear model/2(xdot)
  x/1 -> Landing Gear model/1(x), Gear axes-cg transformation/2("x ")
  massinit/1 -> Gear axes-cg transformation/3(massinit)
  Gear axes-cg transformation/1(FMt) -> Fmt/1
  zero/1 -> Switch/1
  Landing Gear model/1(Forces and Moments) -> Switch/3
  Switch/1 -> Gear axes-cg transformation/1(FMt model)
  ua/1 -> gear position/1
  gear position/1 -> Switch/2
  terr elev/1 -> Landing Gear model/3(terrain elevation)

== system c_citation/Cessna Citation 500/Citation model DASMAT/AIRCRAFT MODEL/OBSERVATIONS ==
  note: Modified by Alex : Flight-Path Subsystem from Ac_mod instead of Ac_modpc
  x : Inport
  xdot : Inport  Port=2
  yuvw : Inport  Port=3
  FMtot : Inport  Port=4
  FMa : Inport  Port=5
  Fgr : Inport  Port=6
  massinit : Inport  Port=7
  yatm : Inport  Port=8
  Acceleration : Subsystem
  Energy : Subsystem
  Flight-Path : Subsystem
  yacc : Outport  VectorParamsAs1DForOutWhenUnconnected=off
  yfp : Outport  Port=2  VectorParamsAs1DForOutWhenUnconnected=off
  ys : Outport  Port=3  VectorParamsAs1DForOutWhenUnconnected=off
  wires:
  yuvw/1 -> Flight-Path/3(yuvw)
  Flight-Path/1(yfp) -> yfp/1
  Energy/1(ys) -> ys/1
  Acceleration/1(yacc) -> yacc/1
  FMa/1 -> Acceleration/4(FMa)
  Fgr/1 -> Acceleration/5(Fgr)
  yatm/1 -> Energy/3(yatm)
  FMtot/1 -> Acceleration/3(FMtot)
  Acceleration/2(acc earth) -> Flight-Path/4(acc earth)
  x/1 -> Flight-Path/1(x), Energy/1(x), Acceleration/1(x)
  xdot/1 -> Flight-Path/2(xdot), Energy/2(xdot), Acceleration/2(xdot)
  massinit/1 -> Acceleration/6(massinit)

== system c_citation/Cessna Citation 500/Citation model DASMAT/AIRCRAFT MODEL/WIND//TURBULENCE ==
  "x " : Inport
  Logarithmic Wind model : Subsystem
  Mux : Mux  Inputs=[12 3]
  Vwind transformation : S-Function  FunctionName=ac_axes  Parameters=3  SFunctionDeploymentMode=off  EnableBusSupport=off
  wind : Outport  VectorParamsAs1DForOutWhenUnconnected=off
  wires:
  Mux/1 -> Vwind transformation/1
  Vwind transformation/1 -> wind/1
  "x "/1 -> Mux/1, Logarithmic Wind model/1(In1)
  Logarithmic Wind model/1(Out1) -> Mux/2

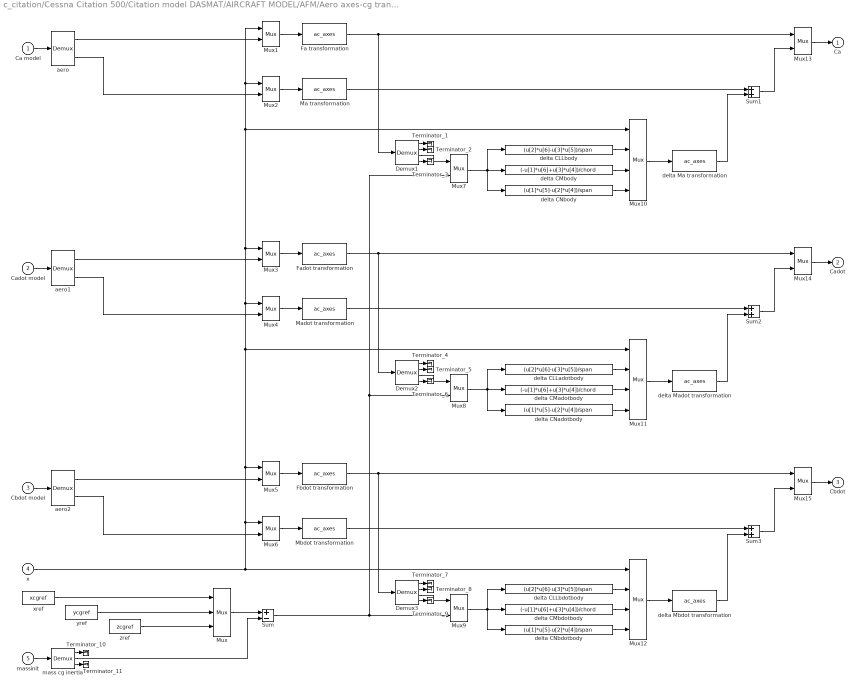
== system c_citation/Cessna Citation 500/Citation model DASMAT/AIRCRAFT MODEL/AFM/Aero axes-cg transformation ==
  Ca model : Inport
  Cadot model : Inport  Port=2
  Cbdot model : Inport  Port=3
  "x " : Inport  Port=4
  massinit : Inport  Port=5
  Demux1 : Demux  Outputs=[3 3 3 3]
      settings: DisplayOption=none
  Demux2 : Demux  Outputs=[3 3 3 3]
      settings: DisplayOption=none
  Demux3 : Demux  Outputs=[3 3 3 3]
      settings: DisplayOption=none
  Fa transformation : S-Function  FunctionName=ac_axes  Parameters=axes_CFMaero  SFunctionDeploymentMode=off  EnableBusSupport=off
  Fadot transformation : S-Function  FunctionName=ac_axes  Parameters=axes_CFMaero  SFunctionDeploymentMode=off  EnableBusSupport=off
  Fbdot transformation : S-Function  FunctionName=ac_axes  Parameters=axes_CFMaero  SFunctionDeploymentMode=off  EnableBusSupport=off
  Ma transformation : S-Function  FunctionName=ac_axes  Parameters=axes_CFMaero  SFunctionDeploymentMode=off  EnableBusSupport=off
  Madot transformation : S-Function  FunctionName=ac_axes  Parameters=axes_CFMaero  SFunctionDeploymentMode=off  EnableBusSupport=off
  Mbdot transformation : S-Function  FunctionName=ac_axes  Parameters=axes_CFMaero  SFunctionDeploymentMode=off  EnableBusSupport=off
  Mux : Mux  Inputs=3
  Mux{1..6} (6 alike) : Mux  Inputs=[12 3]
  Mux10 : Mux  Inputs=[12 1 1 1]
  Mux11 : Mux  Inputs=[12 1 1 1]
  Mux12 : Mux  Inputs=[12 1 1 1]
  Mux13 : Mux  Inputs=[12 12]
  Mux14 : Mux  Inputs=[12 12]
  Mux15 : Mux  Inputs=[12 12]
  Mux7 : Mux  Inputs=[3 3]
  Mux8 : Mux  Inputs=[3 3]
  Mux9 : Mux  Inputs=[3 3]
  Sum : Sum  Inputs=+-  InputSameDT=on  SaturateOnIntegerOverflow=on  OutDataTypeStr=Inherit: Same as first input
  Sum1 : Sum  InputSameDT=on  SaturateOnIntegerOverflow=on  OutDataTypeStr=Inherit: Same as first input
  Sum2 : Sum  InputSameDT=on  SaturateOnIntegerOverflow=on  OutDataTypeStr=Inherit: Same as first input
  Sum3 : Sum  InputSameDT=on  SaturateOnIntegerOverflow=on  OutDataTypeStr=Inherit: Same as first input
  Terminator_{1..11} (11 alike) : Terminator
  aero : Demux  Outputs=[3 3]
      settings: DisplayOption=none
  aero1 : Demux  Outputs=[3 3]
      settings: DisplayOption=none
  aero2 : Demux  Outputs=[3 3]
      settings: DisplayOption=none
  delta CLLadotbody : Fcn  Expr=(u[2]*u[6]-u[3]*u[5])/span
  delta CLLbdotbody : Fcn  Expr=(u[2]*u[6]-u[3]*u[5])/span
  delta CLLbody : Fcn  Expr=(u[2]*u[6]-u[3]*u[5])/span
  delta CMadotbody : Fcn  Expr=(-u[1]*u[6]+u[3]*u[4])/chord
  delta CMbdotbody : Fcn  Expr=(-u[1]*u[6]+u[3]*u[4])/chord
  delta CMbody : Fcn  Expr=(-u[1]*u[6]+u[3]*u[4])/chord
  delta CNadotbody : Fcn  Expr=(u[1]*u[5]-u[2]*u[4])/span
  delta CNbdotbody : Fcn  Expr=(u[1]*u[5]-u[2]*u[4])/span
  delta CNbody : Fcn  Expr=(u[1]*u[5]-u[2]*u[4])/span
  delta Ma transformation : S-Function  FunctionName=ac_axes  Parameters=2  SFunctionDeploymentMode=off  EnableBusSupport=off
  delta Madot transformation : S-Function  FunctionName=ac_axes  Parameters=2  SFunctionDeploymentMode=off  EnableBusSupport=off
  delta Mbdot transformation : S-Function  FunctionName=ac_axes  Parameters=2  SFunctionDeploymentMode=off  EnableBusSupport=off
  mass cg inertia : Demux  Outputs=[1 3 4]
      settings: DisplayOption=none
  xref : Constant  Value=xcgref
  yref : Constant  Value=ycgref
  zref : Constant  Value=zcgref
  Ca : Outport  VectorParamsAs1DForOutWhenUnconnected=off
  Cadot : Outport  Port=2  VectorParamsAs1DForOutWhenUnconnected=off
  Cbdot : Outport  Port=3  VectorParamsAs1DForOutWhenUnconnected=off
  wires:
  mass cg inertia/3 -> Terminator_11/1
  mass cg inertia/1 -> Terminator_10/1
  Demux3/4 -> Terminator_9/1
  Demux3/2 -> Terminator_8/1
  Demux3/1 -> Terminator_7/1
  Demux2/4 -> Terminator_6/1
  Demux2/2 -> Terminator_5/1
  Demux2/1 -> Terminator_4/1
  Demux1/4 -> Terminator_3/1
  Demux1/2 -> Terminator_2/1
  Demux1/1 -> Terminator_1/1
  aero1/1 -> Mux3/2
  Cadot model/1 -> aero1/1
  aero1/2 -> Mux4/2
  Ca model/1 -> aero/1
  massinit/1 -> mass cg inertia/1
  aero/1 -> Mux1/2
  xref/1 -> Mux/1
  yref/1 -> Mux/2
  zref/1 -> Mux/3
  mass cg inertia/2 -> Sum/2
  Mux/1 -> Sum/1
  Fa transformation/1 -> Demux1/1, Mux13/1
  Mux7/1 -> delta CLLbody/1, delta CNbody/1, delta CMbody/1
  delta CLLbody/1 -> Mux10/2
  delta CMbody/1 -> Mux10/3
  delta CNbody/1 -> Mux10/4
  Mux10/1 -> delta Ma transformation/1
  Ma transformation/1 -> Sum1/1
  Sum1/1 -> Mux13/2
  Mux13/1 -> Ca/1
  Mux1/1 -> Fa transformation/1
  Mux3/1 -> Fadot transformation/1
  Mux14/1 -> Cadot/1
  Sum2/1 -> Mux14/2
  Madot transformation/1 -> Sum2/1
  Mux12/1 -> delta Mbdot transformation/1
  delta CNbdotbody/1 -> Mux12/4
  delta CMbdotbody/1 -> Mux12/3
  delta CLLbdotbody/1 -> Mux12/2
  Mux9/1 -> delta CLLbdotbody/1, delta CNbdotbody/1, delta CMbdotbody/1
  Mux4/1 -> Madot transformation/1
  Mux2/1 -> Ma transformation/1
  aero/2 -> Mux2/2
  delta Ma transformation/1 -> Sum1/2
  Demux1/3 -> Mux7/1
  Demux3/3 -> Mux9/1
  Demux2/3 -> Mux8/1
  Mux11/1 -> delta Madot transformation/1
  delta CNadotbody/1 -> Mux11/4
  delta CMadotbody/1 -> Mux11/3
  delta CLLadotbody/1 -> Mux11/2
  Mux8/1 -> delta CLLadotbody/1, delta CNadotbody/1, delta CMadotbody/1
  Fadot transformation/1 -> Demux2/1, Mux14/1
  delta Madot transformation/1 -> Sum2/2
  Sum/1 -> Mux8/2, Mux7/2, Mux9/2
  Mux6/1 -> Mbdot transformation/1
  Mux5/1 -> Fbdot transformation/1
  aero2/2 -> Mux6/2
  Cbdot model/1 -> aero2/1
  aero2/1 -> Mux5/2
  "x "/1 -> Mux4/1, Mux3/1, Mux2/1, Mux1/1, Mux10/1, Mux11/1, Mux5/1, Mux6/1, Mux12/1
  Mbdot transformation/1 -> Sum3/1
  Fbdot transformation/1 -> Demux3/1, Mux15/1
  Sum3/1 -> Mux15/2
  delta Mbdot transformation/1 -> Sum3/2
  Mux15/1 -> Cbdot/1

== system c_citation/Cessna Citation 500/Citation model DASMAT/AIRCRAFT MODEL/AFM/Aeromod ==
  x : Inport
  ua : Inport  Port=2
  massinit : Inport  Port=3
  yad1 : Inport  Port=4
  yad2 : Inport  Port=5
  gust : Inport  Port=6
  yatm : Inport  Port=7
  Demux : Demux  Outputs=[6 6 6 6]
      settings: DisplayOption=none
  Mux1 : Mux  Inputs=24
  SubSystem : Subsystem
  cg selector : Selector  IndexOptions=Index vector (dialog)  Indices=[2 3 4]  OutputSizes=1
  Ca : Outport  VectorParamsAs1DForOutWhenUnconnected=off
  Cadot : Outport  Port=2  VectorParamsAs1DForOutWhenUnconnected=off
  Cbdot : Outport  Port=3  VectorParamsAs1DForOutWhenUnconnected=off
  Cag : Outport  Port=4  VectorParamsAs1DForOutWhenUnconnected=off
  wires:
  Mux1/1 -> Demux/1
  Demux/1 -> Ca/1
  Demux/2 -> Cadot/1
  Demux/3 -> Cbdot/1
  Demux/4 -> Cag/1
  SubSystem/2(CY) -> Mux1/2
  SubSystem/3(CZ) -> Mux1/3
  SubSystem/5(CM) -> Mux1/5
  SubSystem/6(CN) -> Mux1/6
  SubSystem/8(CYadot) -> Mux1/8
  SubSystem/9(CZadot) -> Mux1/9
  SubSystem/11(CMadot) -> Mux1/11
  SubSystem/12(CNadot) -> Mux1/12
  SubSystem/14(CYbdot) -> Mux1/14
  SubSystem/15(CZbdot) -> Mux1/15
  SubSystem/17(CMbdot) -> Mux1/17
  SubSystem/18(CNbdot) -> Mux1/18
  SubSystem/20(CYg) -> Mux1/20
  SubSystem/21(CZg) -> Mux1/21
  SubSystem/23(CMg) -> Mux1/23
  SubSystem/24(CNg) -> Mux1/24
  SubSystem/22(CLLg) -> Mux1/22
  SubSystem/19(CXg) -> Mux1/19
  SubSystem/16(CLLbdot) -> Mux1/16
  SubSystem/13(CXbdot) -> Mux1/13
  SubSystem/10(CLLadot) -> Mux1/10
  SubSystem/7(CXadot) -> Mux1/7
  SubSystem/4(CLL) -> Mux1/4
  SubSystem/1(CX) -> Mux1/1
  massinit/1 -> cg selector/1
  yad1/1 -> SubSystem/4(yad1)
  gust/1 -> SubSystem/6(gust)
  yad2/1 -> SubSystem/5(yad2)
  ua/1 -> SubSystem/2(ua)
  x/1 -> SubSystem/1(x)
  cg selector/1 -> SubSystem/3(cg)
  yatm/1 -> SubSystem/7(yatm)
